simulink model "nonlinear_ADRC"  (R2018a)
settings: Solver=FixedStepAuto  StartTime=0.0  StopTime=60  FixedStep=0.1  RelTol=1e-3
InitFcn:
  | r = 20;
  | delta = 0.25;
  | alpha1 = 0.75;
  | alpha2 = 1.25;
  | b = 0.5;
  | s_cl = 0.2;
  | s_eso = 3 * s_cl;
  | kp = s_cl^2;
  | kd = 2 * s_cl;
  | beta = [3 * s_eso 3 * s_eso^2 s_eso^3];
undefined symbols (not defined in the file or in its folder): As, B1, B2, Cs
settings Model: Creator=leony  LastModifiedBy=leony
settings SolverCC: ZeroCrossAlgorithm=Adaptive
settings DebuggingCC: MaxConsecutiveZCsMsg=none  IgnoredZcDiagnostic=none

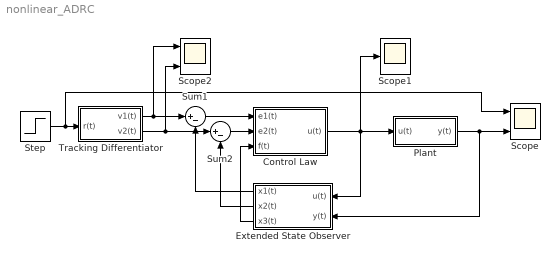
== system nonlinear_ADRC ==
  Control Law : Subsystem
  Extended State Observer : Subsystem
  Plant : Subsystem
  Scope : Scope  NumInputPorts=2
  Scope1 : Scope
  Scope2 : Scope  NumInputPorts=2
  Step : Step  SampleTime=0
  Sum1 : Sum  Inputs=|+-
  Sum2 : Sum  Inputs=|+-
  Tracking Differentiator : Subsystem
  wires:
  Tracking Differentiator/1(v1(t)) -> Scope2/1, Sum1/1
  Extended State Observer/1(x1(t)) -> Sum1/2
  Extended State Observer/2(x2(t)) -> Sum2/2
  Sum1/1 -> Control Law/1(e1(t))
  Sum2/1 -> Control Law/2(e2(t))
  Extended State Observer/3(x3(t)) -> Control Law/3(f(t))
  Control Law/1(u(t)) -> Scope1/1, Plant/1(u(t)), Extended State Observer/1(u(t))
  Plant/1(y(t)) -> Scope/2, Extended State Observer/2(y(t))
  Step/1 -> Scope/1, Tracking Differentiator/1(r(t))
  Tracking Differentiator/2(v2(t)) -> Scope2/2, Sum2/1

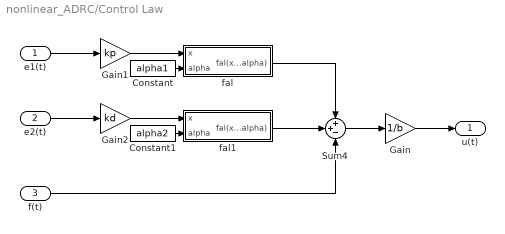
== system nonlinear_ADRC/Control Law ==
  e1(t) : Inport
  e2(t) : Inport  Port=2
  f(t) : Inport  Port=3
  Constant : Constant  Value=alpha1
  Constant1 : Constant  Value=alpha2
  Gain : Gain  Gain=1/b
  Gain1 : Gain  Gain=kp
  Gain2 : Gain  Gain=kd
  Sum4 : Sum  Inputs=++-
  fal : Subsystem
  fal1 : Subsystem
  u(t) : Outport
  wires:
  Sum4/1 -> Gain/1
  Constant1/1 -> fal1/2(alpha)
  Constant/1 -> fal/2(alpha)
  Gain/1 -> u(t)/1
  f(t)/1 -> Sum4/3
  Gain1/1 -> fal/1(x)
  e1(t)/1 -> Gain1/1
  Gain2/1 -> fal1/1(x)
  e2(t)/1 -> Gain2/1
  fal1/1("fal(x, alpha)") -> Sum4/2
  fal/1("fal(x, alpha)") -> Sum4/1

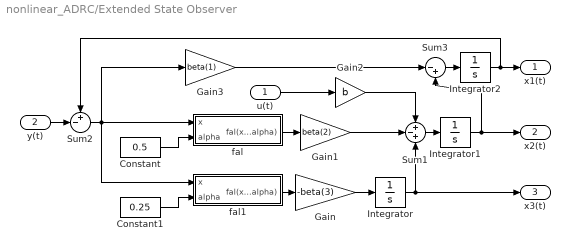
== system nonlinear_ADRC/Extended State Observer ==
  u(t) : Inport
  y(t) : Inport  Port=2
  Constant : Constant  Value=0.5
  Constant1 : Constant  Value=0.25
  Gain : Gain  Gain=-beta(3)
  Gain1 : Gain  Gain=beta(2)
  Gain2 : Gain  Gain=b
  Gain3 : Gain  Gain=beta(1)
  Integrator : Integrator
  Integrator1 : Integrator
  Integrator2 : Integrator
  Sum1 : Sum  Inputs=+-+
  Sum2 : Sum  Inputs=+-|
  Sum3 : Sum  Inputs=|-+
  fal : Subsystem
  fal1 : Subsystem
  x1(t) : Outport
  x2(t) : Outport  Port=2
  x3(t) : Outport  Port=3
  wires:
  fal1/1("fal(x, alpha)") -> Gain/1
  fal/1("fal(x, alpha)") -> Gain1/1
  Constant1/1 -> fal1/2(alpha)
  Integrator2/1 -> Sum2/1, x1(t)/1
  Sum1/1 -> Integrator1/1
  Gain/1 -> Integrator/1
  Integrator/1 -> Sum1/3, x3(t)/1
  Gain1/1 -> Sum1/2
  Integrator1/1 -> Sum3/2, x2(t)/1
  Sum2/1 -> Gain3/1, fal/1(x), fal1/1(x)
  Constant/1 -> fal/2(alpha)
  Sum3/1 -> Integrator2/1
  y(t)/1 -> Sum2/2
  u(t)/1 -> Gain2/1
  Gain2/1 -> Sum1/1
  Gain3/1 -> Sum3/1

== system nonlinear_ADRC/Plant ==
  u(t) : Inport
  "Two Mass-Spring System " : Subsystem
  y(t) : Outport
  wires:
  "Two Mass-Spring System "/1(y(t)) -> y(t)/1
  u(t)/1 -> "Two Mass-Spring System "/1(f(t))

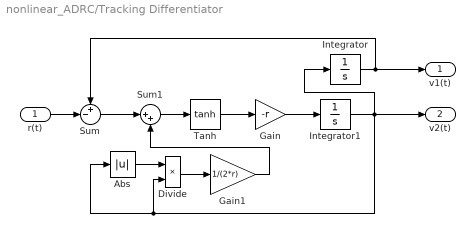
== system nonlinear_ADRC/Tracking Differentiator ==
  r(t) : Inport
  Abs : Abs
  Divide : Product  Inputs=**
  Gain : Gain  Gain=-r
  Gain1 : Gain  Gain=1/(2*r)
  Integrator : Integrator
  Integrator1 : Integrator
  Sum : Sum  Inputs=+-|
  Sum1 : Sum  Inputs=|++
  Tanh : Trigonometry  Operator=tanh
  v1(t) : Outport
  v2(t) : Outport  Port=2
  wires:
  r(t)/1 -> Sum/2
  Integrator1/1 -> Abs/1, Divide/2, v2(t)/1, Integrator/1
  Integrator/1 -> Sum/1, v1(t)/1
  Abs/1 -> Divide/1
  Divide/1 -> Gain1/1
  Gain1/1 -> Sum1/2
  Sum/1 -> Sum1/1
  Sum1/1 -> Tanh/1
  Tanh/1 -> Gain/1
  Gain/1 -> Integrator1/1

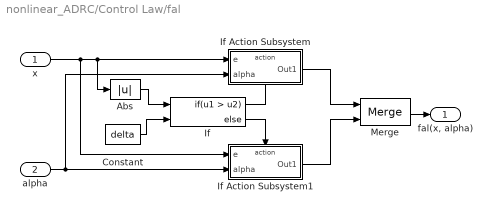
== system nonlinear_ADRC/Control Law/fal ==
  x : Inport
  alpha : Inport  Port=2
  Abs : Abs
  Constant : Constant  Value=delta
  If : If  NumInputs=2  IfExpression=u1 > u2
  If Action Subsystem : Subsystem  TreatAsAtomicUnit=on
  If Action Subsystem1 : Subsystem  TreatAsAtomicUnit=on
  Merge : Merge
  "fal(x, alpha)" : Outport
  wires:
  x/1 -> If Action Subsystem1/1(e), Abs/1, If Action Subsystem/1(e)
  If/1 -> If Action Subsystem/Action
  If Action Subsystem1/1(Out1) -> Merge/2
  Abs/1 -> If/1
  Merge/1 -> "fal(x, alpha)"/1
  Constant/1 -> If/2
  If/2 -> If Action Subsystem1/Action
  If Action Subsystem/1(Out1) -> Merge/1
  alpha/1 -> If Action Subsystem/2(alpha), If Action Subsystem1/2(alpha)

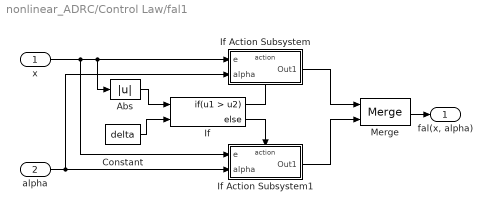
== system nonlinear_ADRC/Control Law/fal1 ==
  x : Inport
  alpha : Inport  Port=2
  Abs : Abs
  Constant : Constant  Value=delta
  If : If  NumInputs=2  IfExpression=u1 > u2
  If Action Subsystem : Subsystem  TreatAsAtomicUnit=on
  If Action Subsystem1 : Subsystem  TreatAsAtomicUnit=on
  Merge : Merge
  "fal(x, alpha)" : Outport
  wires:
  x/1 -> If Action Subsystem1/1(e), Abs/1, If Action Subsystem/1(e)
  If/1 -> If Action Subsystem/Action
  If Action Subsystem1/1(Out1) -> Merge/2
  Abs/1 -> If/1
  Merge/1 -> "fal(x, alpha)"/1
  Constant/1 -> If/2
  If/2 -> If Action Subsystem1/Action
  If Action Subsystem/1(Out1) -> Merge/1
  alpha/1 -> If Action Subsystem/2(alpha), If Action Subsystem1/2(alpha)

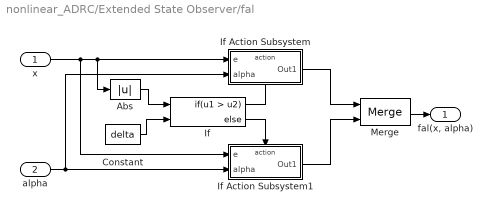
== system nonlinear_ADRC/Extended State Observer/fal ==
  x : Inport
  alpha : Inport  Port=2
  Abs : Abs
  Constant : Constant  Value=delta
  If : If  NumInputs=2  IfExpression=u1 > u2
  If Action Subsystem : Subsystem  TreatAsAtomicUnit=on
  If Action Subsystem1 : Subsystem  TreatAsAtomicUnit=on
  Merge : Merge
  "fal(x, alpha)" : Outport
  wires:
  x/1 -> If Action Subsystem1/1(e), Abs/1, If Action Subsystem/1(e)
  If/1 -> If Action Subsystem/Action
  If Action Subsystem1/1(Out1) -> Merge/2
  Abs/1 -> If/1
  Merge/1 -> "fal(x, alpha)"/1
  Constant/1 -> If/2
  If/2 -> If Action Subsystem1/Action
  If Action Subsystem/1(Out1) -> Merge/1
  alpha/1 -> If Action Subsystem/2(alpha), If Action Subsystem1/2(alpha)

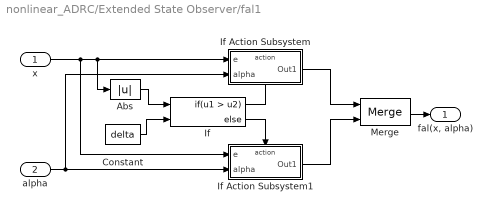
== system nonlinear_ADRC/Extended State Observer/fal1 ==
  x : Inport
  alpha : Inport  Port=2
  Abs : Abs
  Constant : Constant  Value=delta
  If : If  NumInputs=2  IfExpression=u1 > u2
  If Action Subsystem : Subsystem  TreatAsAtomicUnit=on
  If Action Subsystem1 : Subsystem  TreatAsAtomicUnit=on
  Merge : Merge
  "fal(x, alpha)" : Outport
  wires:
  x/1 -> If Action Subsystem1/1(e), Abs/1, If Action Subsystem/1(e)
  If/1 -> If Action Subsystem/Action
  If Action Subsystem1/1(Out1) -> Merge/2
  Abs/1 -> If/1
  Merge/1 -> "fal(x, alpha)"/1
  Constant/1 -> If/2
  If/2 -> If Action Subsystem1/Action
  If Action Subsystem/1(Out1) -> Merge/1
  alpha/1 -> If Action Subsystem/2(alpha), If Action Subsystem1/2(alpha)

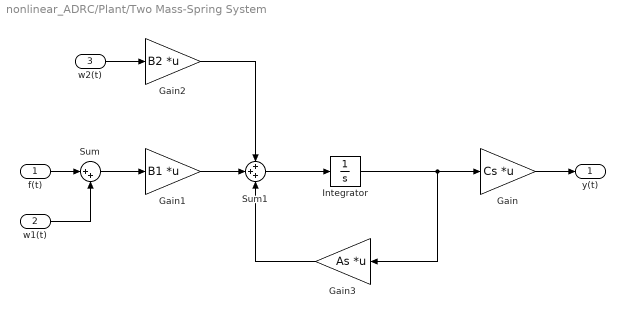
== system nonlinear_ADRC/Plant/Two Mass-Spring System  ==
  f(t) : Inport
  w1(t) : Inport  Port=2
  w2(t) : Inport  Port=3
  Gain : Gain  Gain=Cs  Multiplication=Matrix(K*u) (u vector)
  Gain1 : Gain  Gain=B1  Multiplication=Matrix(K*u) (u vector)
  Gain2 : Gain  Gain=B2  Multiplication=Matrix(K*u) (u vector)
  Gain3 : Gain  Gain=As  Multiplication=Matrix(K*u) (u vector)
  Integrator : Integrator
  Sum : Sum  Inputs=|++
  Sum1 : Sum  Inputs=+++
  y(t) : Outport
  wires:
  Gain/1 -> y(t)/1
  Integrator/1 -> Gain3/1, Gain/1
  f(t)/1 -> Sum/1
  Sum/1 -> Gain1/1
  Gain1/1 -> Sum1/2
  Gain3/1 -> Sum1/3
  Sum1/1 -> Integrator/1
  Gain2/1 -> Sum1/1
  w2(t)/1 -> Gain2/1
  w1(t)/1 -> Sum/2

== system nonlinear_ADRC/Control Law/fal/If Action Subsystem ==
  e : Inport
  alpha : Inport  Port=2
  Action Port : ActionPort  PropagateVarSize=During execution  ActionType=then
  Abs : Abs
  Power : Math  Operator=pow  SaturateOnIntegerOverflow=on
  Product : Product
  Sign : Signum
  Out1 : Outport
  wires:
  Abs/1 -> Power/1
  alpha/1 -> Power/2
  e/1 -> Sign/1, Abs/1
  Sign/1 -> Product/1
  Power/1 -> Product/2
  Product/1 -> Out1/1

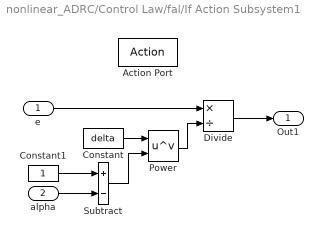
== system nonlinear_ADRC/Control Law/fal/If Action Subsystem1 ==
  e : Inport
  alpha : Inport  Port=2
  Action Port : ActionPort  PropagateVarSize=During execution  ActionType=else
  Constant : Constant  Value=delta
  Constant1 : Constant
  Divide : Product  Inputs=*/
  Power : Math  Operator=pow  SaturateOnIntegerOverflow=on
  Subtract : Sum  Inputs=+-
  Out1 : Outport
  wires:
  e/1 -> Divide/1
  Divide/1 -> Out1/1
  Constant/1 -> Power/1
  Constant1/1 -> Subtract/1
  alpha/1 -> Subtract/2
  Subtract/1 -> Power/2
  Power/1 -> Divide/2

== system nonlinear_ADRC/Control Law/fal1/If Action Subsystem ==
  e : Inport
  alpha : Inport  Port=2
  Action Port : ActionPort  PropagateVarSize=During execution  ActionType=then
  Abs : Abs
  Power : Math  Operator=pow  SaturateOnIntegerOverflow=on
  Product : Product
  Sign : Signum
  Out1 : Outport
  wires:
  Abs/1 -> Power/1
  alpha/1 -> Power/2
  e/1 -> Sign/1, Abs/1
  Sign/1 -> Product/1
  Power/1 -> Product/2
  Product/1 -> Out1/1

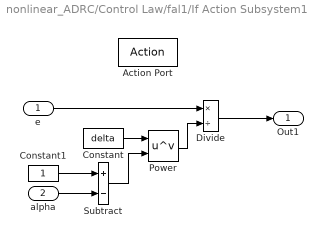
== system nonlinear_ADRC/Control Law/fal1/If Action Subsystem1 ==
  e : Inport
  alpha : Inport  Port=2
  Action Port : ActionPort  PropagateVarSize=During execution  ActionType=else
  Constant : Constant  Value=delta
  Constant1 : Constant
  Divide : Product  Inputs=*/
  Power : Math  Operator=pow  SaturateOnIntegerOverflow=on
  Subtract : Sum  Inputs=+-
  Out1 : Outport
  wires:
  e/1 -> Divide/1
  Divide/1 -> Out1/1
  Constant/1 -> Power/1
  Constant1/1 -> Subtract/1
  alpha/1 -> Subtract/2
  Subtract/1 -> Power/2
  Power/1 -> Divide/2

== system nonlinear_ADRC/Extended State Observer/fal/If Action Subsystem ==
  e : Inport
  alpha : Inport  Port=2
  Action Port : ActionPort  PropagateVarSize=During execution  ActionType=then
  Abs : Abs
  Power : Math  Operator=pow  SaturateOnIntegerOverflow=on
  Product : Product
  Sign : Signum
  Out1 : Outport
  wires:
  Abs/1 -> Power/1
  alpha/1 -> Power/2
  e/1 -> Sign/1, Abs/1
  Sign/1 -> Product/1
  Power/1 -> Product/2
  Product/1 -> Out1/1

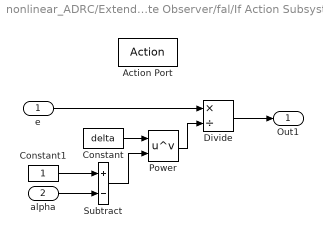
== system nonlinear_ADRC/Extended State Observer/fal/If Action Subsystem1 ==
  e : Inport
  alpha : Inport  Port=2
  Action Port : ActionPort  PropagateVarSize=During execution  ActionType=else
  Constant : Constant  Value=delta
  Constant1 : Constant
  Divide : Product  Inputs=*/
  Power : Math  Operator=pow  SaturateOnIntegerOverflow=on
  Subtract : Sum  Inputs=+-
  Out1 : Outport
  wires:
  e/1 -> Divide/1
  Divide/1 -> Out1/1
  Constant/1 -> Power/1
  Constant1/1 -> Subtract/1
  alpha/1 -> Subtract/2
  Subtract/1 -> Power/2
  Power/1 -> Divide/2

== system nonlinear_ADRC/Extended State Observer/fal1/If Action Subsystem ==
  e : Inport
  alpha : Inport  Port=2
  Action Port : ActionPort  PropagateVarSize=During execution  ActionType=then
  Abs : Abs
  Power : Math  Operator=pow  SaturateOnIntegerOverflow=on
  Product : Product
  Sign : Signum
  Out1 : Outport
  wires:
  Abs/1 -> Power/1
  alpha/1 -> Power/2
  e/1 -> Sign/1, Abs/1
  Sign/1 -> Product/1
  Power/1 -> Product/2
  Product/1 -> Out1/1

== system nonlinear_ADRC/Extended State Observer/fal1/If Action Subsystem1 ==
  e : Inport
  alpha : Inport  Port=2
  Action Port : ActionPort  PropagateVarSize=During execution  ActionType=else
  Constant : Constant  Value=delta
  Constant1 : Constant
  Divide : Product  Inputs=*/
  Power : Math  Operator=pow  SaturateOnIntegerOverflow=on
  Subtract : Sum  Inputs=+-
  Out1 : Outport
  wires:
  e/1 -> Divide/1
  Divide/1 -> Out1/1
  Constant/1 -> Power/1
  Constant1/1 -> Subtract/1
  alpha/1 -> Subtract/2
  Subtract/1 -> Power/2
  Power/1 -> Divide/2
